simulink model "soru2d1"  (R2019a)
settings: Solver=VariableStepAuto  StartTime=0.0  StopTime=1000  RelTol=1e-3
settings Model: Creator=handeyildirim  LastModifiedBy=handeyildirim

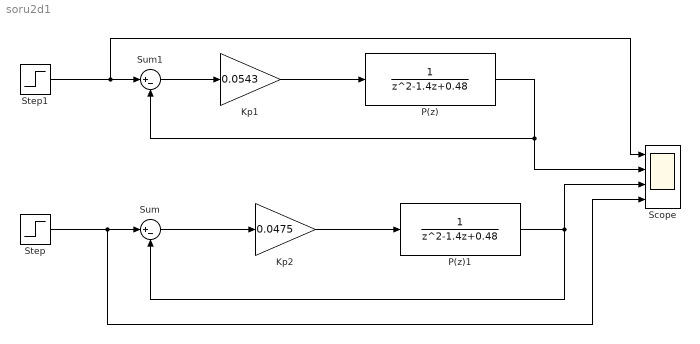
== system soru2d1 ==
  Kp1 : Gain  Gain=0.0543
  Kp2 : Gain  Gain=0.0475
  P(z) : DiscreteTransferFcn  Denominator=[1 -1.4 0.48]  SampleTime=1
  P(z)1 : DiscreteTransferFcn  Denominator=[1 -1.4 0.48]  SampleTime=1
  Scope : Scope  NumInputPorts=4
  Step : Step  SampleTime=1
  Step1 : Step  SampleTime=1
  Sum : Sum  Inputs=|+-
  Sum1 : Sum  Inputs=|+-
  wires:
  P(z)1/1 -> Scope/3, Sum/2
  Sum/1 -> Kp2/1
  Kp2/1 -> P(z)1/1
  Step/1 -> Scope/4, Sum/1
  Step1/1 -> Scope/1, Sum1/1
  P(z)/1 -> Scope/2, Sum1/2
  Kp1/1 -> P(z)/1
  Sum1/1 -> Kp1/1
